simulink model "uav_open_loop"  (R2024b)
settings: Solver=VariableStepAuto  StartTime=0.0  StopTime=10  RelTol=1e-3
undefined symbols (not defined in the file): g, kf, km, L, m, omega_hover, P, tau_propeller
settings Model: Creator=erhan  LastModifiedBy=erhan

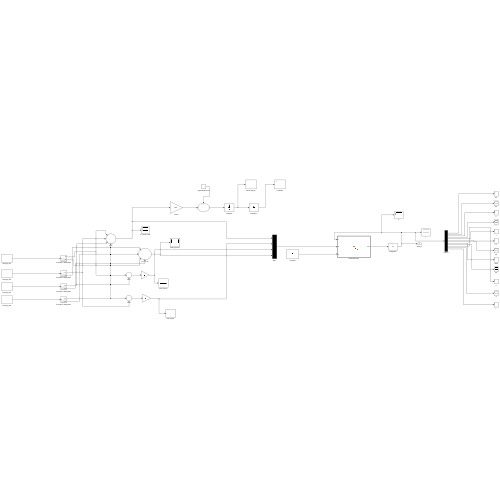
[thumbnail: Simulink's stored preview of the top-level diagram]
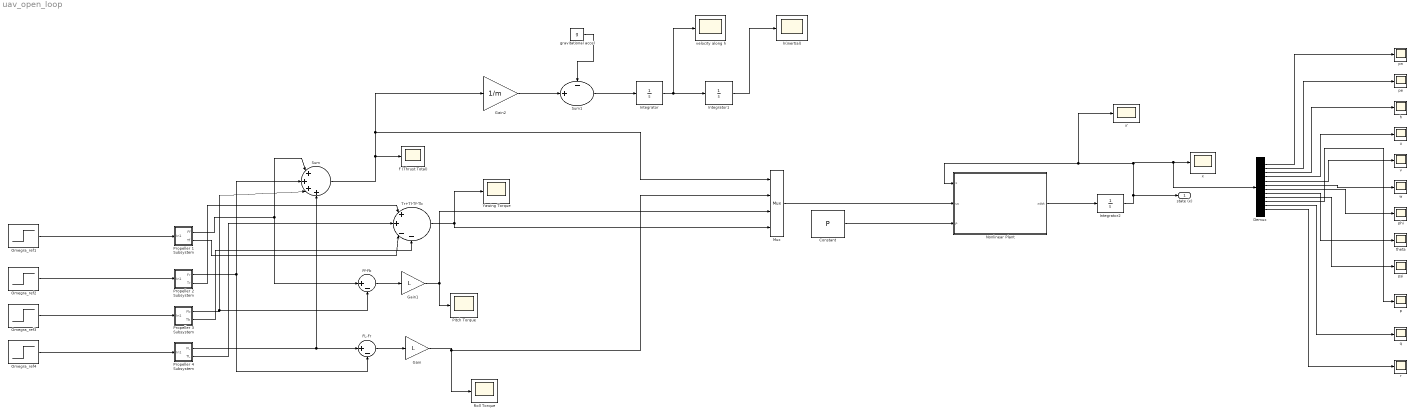
== system uav_open_loop ==
  Constant : Constant  Value=P
  Demux : Demux  Outputs=12
  F (Thrust Total) : Scope
  FL-Fr : Sum  Inputs=|+-
  Ff-Fb : Sum  Inputs=|+-
  Gain : Gain  Gain=L
  Gain1 : Gain  Gain=L
  Gain2 : Gain  Gain=1/m
  Integrator : Integrator
  Integrator1 : Integrator
  Integrator2 : Integrator  InitialCondition=zeros(12,1)
  Mux : Mux
  Nonlinear Plant : MATLAB Function  TreatAsAtomicUnit=on
  Omegra_ref{1..4} (4 alike) : Step  Time=0  After=omega_hover  SampleTime=0
  Pitch Torque : Scope
  Propeller 1 Subsystem : Subsystem
  Propeller 2 Subsystem : Subsystem
  Propeller 3 Subsystem : Subsystem
  Propeller 4 Subsystem : Subsystem
  Roll Torque : Scope
  Sum : Sum  Inputs=|++++
  Sum1 : Sum  Inputs=-+|
  Tr+Tl-Tf-Tb : Sum  Inputs=|++--
  Yawing Torque : Scope
  gravitational accel : Constant  Value=g
  h : Scope
  h(inertial) : Scope
  p : Scope
  pe : Scope
  phi : Scope
  pn : Scope
  psi : Scope
  q : Scope
  r : Scope
  theta : Scope
  u : Scope
  v : Scope
  "velocity along h " : Scope
  w : Scope
  x : Scope
  x' : Scope
  state (x) : Outport
  wires:
  Omegra_ref1/1 -> Propeller 1 Subsystem/1(In1)
  Omegra_ref2/1 -> Propeller 2 Subsystem/1(In1)
  Omegra_ref3/1 -> Propeller 3 Subsystem/1(In1)
  Omegra_ref4/1 -> Propeller 4 Subsystem/1(In1)
  Propeller 1 Subsystem/1(Ff) -> Ff-Fb/1, Sum/1
  Propeller 2 Subsystem/1(Fr) -> FL-Fr/2, Sum/2
  Propeller 3 Subsystem/1(Fb) -> Ff-Fb/2, Sum/3
  Propeller 4 Subsystem/1(FL) -> Sum/4, FL-Fr/1
  Sum/1 -> Gain2/1, Mux/1, F (Thrust Total)/1
  FL-Fr/1 -> Gain/1
  Gain/1 -> Mux/2, Roll Torque/1
  Ff-Fb/1 -> Gain1/1
  Gain1/1 -> Mux/3, Pitch Torque/1
  Propeller 2 Subsystem/2(Tr) -> Tr+Tl-Tf-Tb/1
  Propeller 4 Subsystem/2(TL) -> Tr+Tl-Tf-Tb/2
  Propeller 1 Subsystem/2(Tf) -> Tr+Tl-Tf-Tb/3
  Propeller 3 Subsystem/2(Tb) -> Tr+Tl-Tf-Tb/4
  Tr+Tl-Tf-Tb/1 -> Mux/4, Yawing Torque/1
  Gain2/1 -> Sum1/2
  gravitational accel/1 -> Sum1/1
  Sum1/1 -> Integrator/1
  Integrator/1 -> "velocity along h "/1, Integrator1/1
  Integrator1/1 -> h(inertial)/1
  Mux/1 -> Nonlinear Plant/2(uc)
  Nonlinear Plant/1(xdot) -> Integrator2/1
  Integrator2/1 -> state (x)/1, Demux/1, x/1, x'/1, Nonlinear Plant/1(x)
  Constant/1 -> Nonlinear Plant/3(P)
  Demux/1 -> pn/1
  Demux/2 -> pe/1
  Demux/3 -> h/1
  Demux/4 -> u/1
  Demux/5 -> v/1
  Demux/6 -> w/1
  Demux/7 -> phi/1
  Demux/8 -> theta/1
  Demux/9 -> psi/1
  Demux/10 -> p/1
  Demux/11 -> q/1
  Demux/12 -> r/1

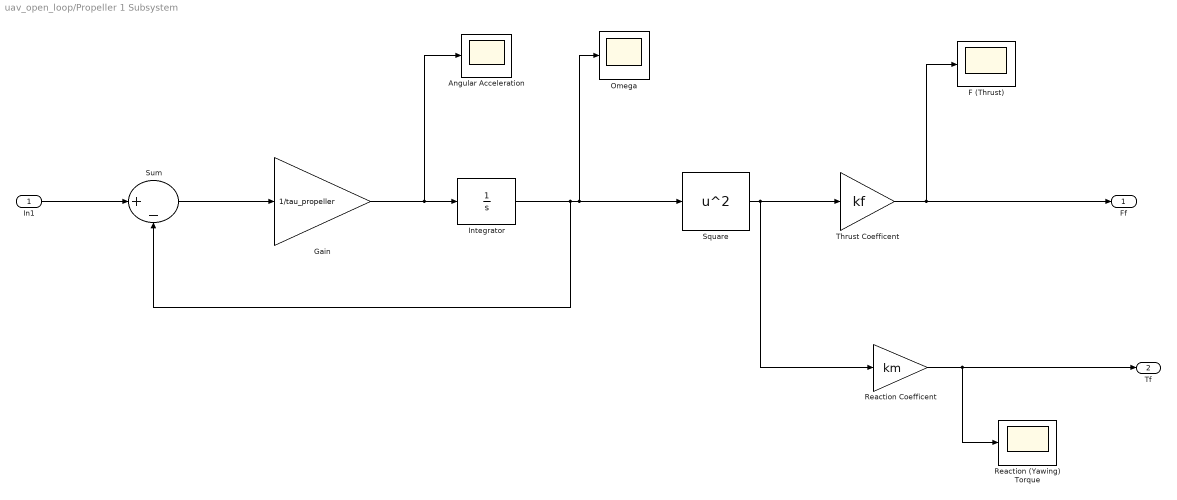
== system uav_open_loop/Propeller 1 Subsystem ==
  In1 : Inport
  Angular Acceleration : Scope
  F (Thrust) : Scope
  Gain : Gain  Gain=1/tau_propeller
  Integrator : Integrator
  Omega : Scope
  Reaction (Yawing) Torque : Scope
  Reaction Coefficent : Gain  Gain=km
  Square : Math  Operator=square
  Sum : Sum  Inputs=|+-
  Thrust Coefficent : Gain  Gain=kf
  Ff : Outport
  Tf : Outport  Port=2
  wires:
  Gain/1 -> Angular Acceleration/1, Integrator/1
  Reaction Coefficent/1 -> Tf/1, Reaction (Yawing) Torque/1
  Square/1 -> Reaction Coefficent/1, Thrust Coefficent/1
  In1/1 -> Sum/1
  Sum/1 -> Gain/1
  Integrator/1 -> Square/1, Omega/1, Sum/2
  Thrust Coefficent/1 -> Ff/1, F (Thrust)/1

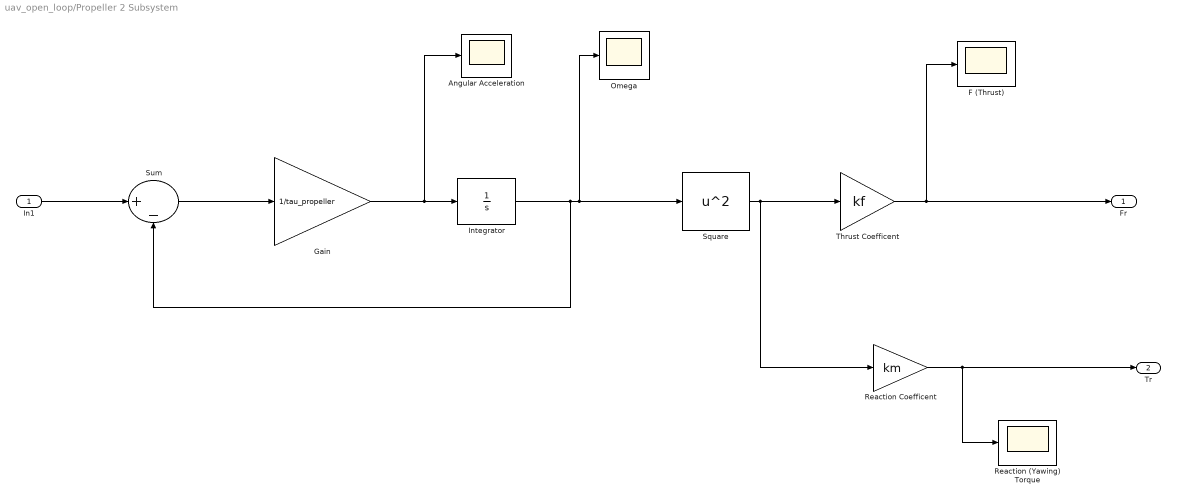
== system uav_open_loop/Propeller 2 Subsystem ==
  In1 : Inport
  Angular Acceleration : Scope
  F (Thrust) : Scope
  Gain : Gain  Gain=1/tau_propeller
  Integrator : Integrator
  Omega : Scope
  Reaction (Yawing) Torque : Scope
  Reaction Coefficent : Gain  Gain=km
  Square : Math  Operator=square
  Sum : Sum  Inputs=|+-
  Thrust Coefficent : Gain  Gain=kf
  Fr : Outport
  Tr : Outport  Port=2
  wires:
  Gain/1 -> Angular Acceleration/1, Integrator/1
  Reaction Coefficent/1 -> Tr/1, Reaction (Yawing) Torque/1
  Square/1 -> Reaction Coefficent/1, Thrust Coefficent/1
  In1/1 -> Sum/1
  Sum/1 -> Gain/1
  Integrator/1 -> Square/1, Omega/1, Sum/2
  Thrust Coefficent/1 -> Fr/1, F (Thrust)/1

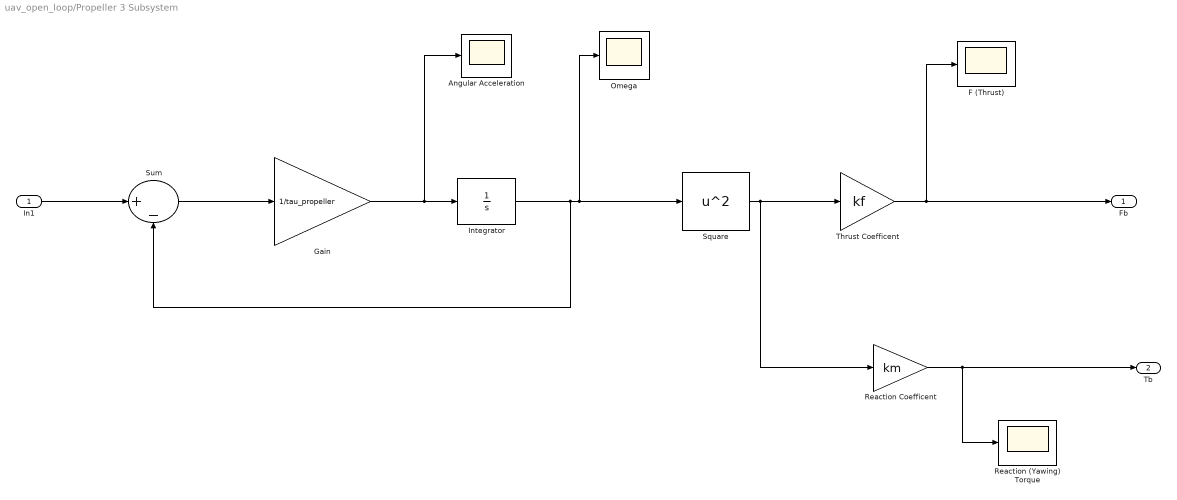
== system uav_open_loop/Propeller 3 Subsystem ==
  In1 : Inport
  Angular Acceleration : Scope
  F (Thrust) : Scope
  Gain : Gain  Gain=1/tau_propeller
  Integrator : Integrator
  Omega : Scope
  Reaction (Yawing) Torque : Scope
  Reaction Coefficent : Gain  Gain=km
  Square : Math  Operator=square
  Sum : Sum  Inputs=|+-
  Thrust Coefficent : Gain  Gain=kf
  Fb : Outport
  Tb : Outport  Port=2
  wires:
  Gain/1 -> Angular Acceleration/1, Integrator/1
  Reaction Coefficent/1 -> Tb/1, Reaction (Yawing) Torque/1
  Square/1 -> Reaction Coefficent/1, Thrust Coefficent/1
  In1/1 -> Sum/1
  Sum/1 -> Gain/1
  Integrator/1 -> Square/1, Omega/1, Sum/2
  Thrust Coefficent/1 -> Fb/1, F (Thrust)/1

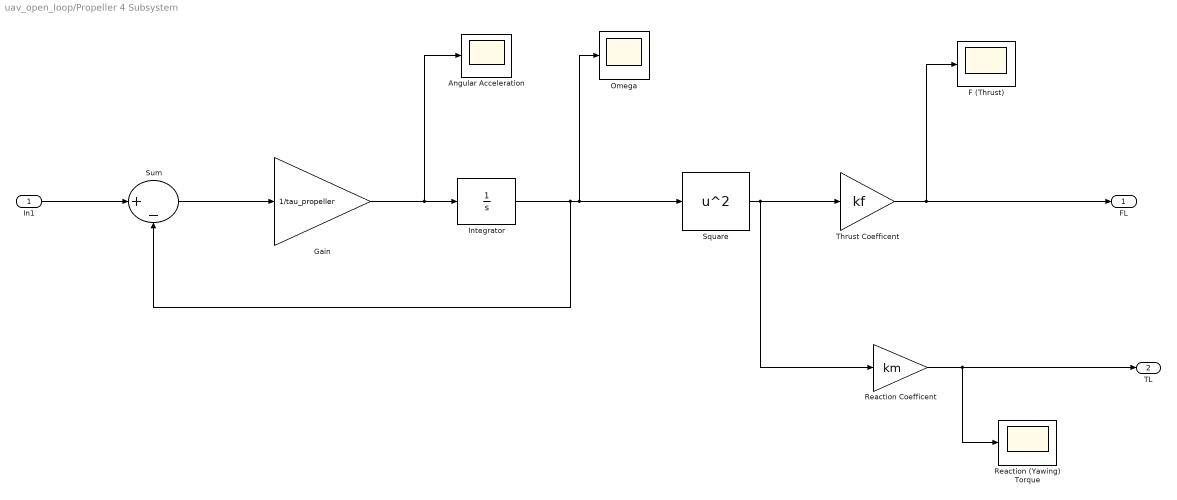
== system uav_open_loop/Propeller 4 Subsystem ==
  In1 : Inport
  Angular Acceleration : Scope
  F (Thrust) : Scope
  Gain : Gain  Gain=1/tau_propeller
  Integrator : Integrator
  Omega : Scope
  Reaction (Yawing) Torque : Scope
  Reaction Coefficent : Gain  Gain=km
  Square : Math  Operator=square
  Sum : Sum  Inputs=|+-
  Thrust Coefficent : Gain  Gain=kf
  FL : Outport
  TL : Outport  Port=2
  wires:
  Gain/1 -> Angular Acceleration/1, Integrator/1
  Reaction Coefficent/1 -> TL/1, Reaction (Yawing) Torque/1
  Square/1 -> Reaction Coefficent/1, Thrust Coefficent/1
  In1/1 -> Sum/1
  Sum/1 -> Gain/1
  Integrator/1 -> Square/1, Omega/1, Sum/2
  Thrust Coefficent/1 -> FL/1, F (Thrust)/1

== matlab function uav_open_loop/Nonlinear Plant ==
  data: x input; xdot output; uc input; P input
function xdot = nonlinearstatespace(x,uc,P)
% Nonlinear quadrotor state-space model
%
% x  = [pn pe h u v w phi theta psi p q r]'
% uc = [F tau_phi tau_theta tau_psi]'
% P  = [m g Jx Jy Jz]'

%% Parameters
m  = P(1);
g  = P(2);
Jx = P(3);
Jy = P(4);
Jz = P(5);

%% Generalized control inputs
F         = uc(1,1);
tau_phi   = uc(2,1);
tau_theta = uc(3,1);
tau_psi   = uc(4,1);

%% State variables
u     = x(4,1);
v     = x(5,1);
w     = x(6,1);
phi   = x(7,1);
theta = x(8,1);
psi   = x(9,1);
p     = x(10,1);
q     = x(11,1);
r     = x(12,1);

%% Useful trigonometric quantities
cphi   = cos(phi);
sphi   = sin(phi);
ctheta = cos(theta);
stheta = sin(theta);
cpsi   = cos(psi);
spsi   = sin(psi);

%% Position kinematics: inertial position rates
pn_dot = ctheta*cpsi*u ...
       + (sphi*stheta*cpsi-cphi*spsi)*v ...
       + (cphi*stheta*cpsi+sphi*spsi)*w;

pe_dot = ctheta*spsi*u ...
       + (sphi*stheta*spsi+cphi*cpsi)*v ...
       + (cphi*stheta*spsi-sphi*cpsi)*w;

h_dot = stheta*u ...
      - sphi*ctheta*v ...
      - cphi*ctheta*w;

%% Translational dynamics in body coordinates
u_dot = r*v-q*w-g*stheta;

v_dot = p*w-r*u+g*ctheta*sphi;

w_dot = q*u-p*v+g*ctheta*cphi-F/m;

%% Euler-angle kinematics
phi_dot = p ...
        + q*sphi*tan(theta) ...
        + r*cphi*tan(theta);

theta_dot = q*cphi-r*sphi;

psi_dot = (q*sphi+r*cphi)/ctheta;

%% Rotational rigid-body dynamics
p_dot = ((Jy-Jz)/Jx)*q*r+tau_phi/Jx;

q_dot = ((Jz-Jx)/Jy)*p*r+tau_theta/Jy;

r_dot = ((Jx-Jy)/Jz)*p*q+tau_psi/Jz;

%% Nonlinear state equation
xdot = [pn_dot;
        pe_dot;
        h_dot;
        u_dot;
        v_dot;
        w_dot;
        phi_dot;
        theta_dot;
        psi_dot;
        p_dot;
        q_dot;
        r_dot];
end
